simulink model "sim_v2"  (R2016b)
settings: Solver=VariableStepAuto  StartTime=0.0  StopTime=tfin  RelTol=1e-3
values from neighbouring files (symbols this model uses):
  ahat_inner_t0 = 0.5*[ahat_in1; ahat_in2]    [sim_script_circle.m]    (also in sim_script_v2.m = [ahat_in1; ahat_in2])
  ahat_outer_t0 = 0.5*[(m+m_p); c_d]    [sim_script_circle.m]    (also in sim_script_v2.m = [(m+m_p); c_d])
  c_d = 4 * 1.225 * 0.32    (= 1.568)    [sim_script_circle.m]    (also in sim_script_v2.m = 0)
  dx0 = xd(1,2)    [sim_script_circle.m]    (also in sim_script_v2.m = states(1,3))
  dz0 = zd(1,2)    [sim_script_circle.m]    (also in sim_script_v2.m = states(1,4))
  g = 9.81    [sim_script_circle.m]    (also in sim_script_v2.m)
  Gamma = 2 * diag([1, 1])    [sim_script_circle.m]    (also in sim_script_v2.m)
  Gamma_out = 0.2 * diag([1, 1])    [sim_script_circle.m]    (also in sim_script_v2.m)
  k_th = 0.2    [sim_script_circle.m]    (also in sim_script_v2.m)
  k_x = 6    [sim_script_circle.m]    (also in sim_script_v2.m)
  k_z = 6    [sim_script_circle.m]    (also in sim_script_v2.m)
  l = 0.5    [sim_script_circle.m]    (also in sim_script_v2.m)
  lambda = 3    [sim_script_circle.m]    (also in sim_script_v2.m)
  lambda_in = 6    [sim_script_circle.m]    (also in sim_script_v2.m)
  m = 3    [sim_script_circle.m]    (also in sim_script_v2.m)
  Phi_th = 0.1    [sim_script_circle.m]    (also in sim_script_v2.m)
  Phi_x = 0.4    [sim_script_circle.m]    (also in sim_script_v2.m)
  Phi_z = 0.4    [sim_script_circle.m]    (also in sim_script_v2.m)
  plan_mass = 1    [sim_script_circle.m]    (also in sim_script_v2.m = 5)
  th0 = -atan2(xd(1,3),zd(1,3)+g)    [sim_script_circle.m]    (also in sim_script_v2.m = -atan2(u(1,1)/(m+m_p),u(1,2)/(m+m_p)+g))
  Tmax = 80    [sim_script_circle.m]    (also in sim_script_v2.m)
  var_rnd = 6    [sim_script_circle.m]    (also in sim_script_v2.m)
  x0 = xd(1,1)    [sim_script_circle.m]    (also in sim_script_v2.m = states(1,1))
  z0 = zd(1,1)    [sim_script_circle.m]    (also in sim_script_v2.m = states(1,2))
libraries: cstblocks x2
settings Model: Creator=ben  LastModifiedBy=ben
settings SolverCC: ZeroCrossControl=EnableAll
settings DataIOCC: SaveOutput=off

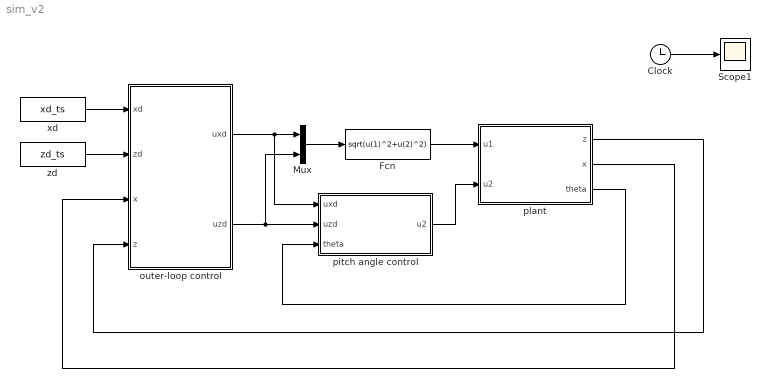
== system sim_v2 ==
  Clock : Clock
      settings: Decimation=2
  Fcn : Fcn  Expr=sqrt(u(1)^2+u(2)^2)
  Mux : Mux  Inputs=2
  Scope1 : Scope
  outer-loop control : Subsystem
  pitch angle control : Subsystem
  plant : Subsystem
  xd : FromWorkspace  VariableName=xd_ts  SampleTime=0
  zd : FromWorkspace  VariableName=zd_ts  SampleTime=0
  wires:
  xd/1 -> outer-loop control/1(xd)
  zd/1 -> outer-loop control/2(zd)
  plant/1(z) -> outer-loop control/4(z)
  plant/2(x) -> outer-loop control/3(x)
  Mux/1 -> Fcn/1
  outer-loop control/1(uxd) -> pitch angle control/1(uxd), Mux/1
  outer-loop control/2(uzd) -> pitch angle control/2(uzd), Mux/2
  Fcn/1 -> plant/1(u1)
  pitch angle control/1(u2) -> plant/2(u2)
  plant/3(theta) -> pitch angle control/3(theta)
  Clock/1 -> Scope1/1

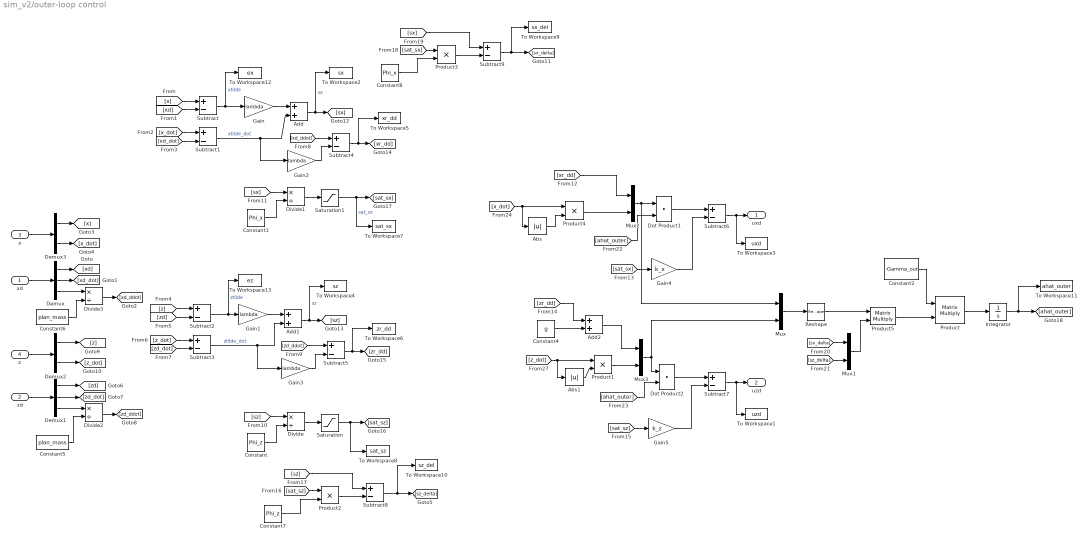
== system sim_v2/outer-loop control ==
  xd : Inport
  zd : Inport  Port=2
  x : Inport  Port=3
  z : Inport  Port=4
  Abs : Abs
  Abs1 : Abs
  Add : Sum
  Add1 : Sum
  Add2 : Sum
  Constant : Constant  Value=Phi_z
  Constant1 : Constant  Value=Phi_x
  Constant2 : Constant  Value=-Gamma_out
  Constant4 : Constant  Value=g
  Constant5 : Constant  Value=plan_mass
  Constant6 : Constant  Value=plan_mass
  Constant7 : Constant  Value=Phi_z
  Constant8 : Constant  Value=Phi_x
  Demux : Demux  Outputs=3
  Demux1 : Demux  Outputs=3
  Demux2 : Demux  Outputs=2
  Demux3 : Demux  Outputs=2
  Divide{,1..3} (4 alike) : Product  Inputs=*/
  Dot Product1 : DotProduct  InputSameDT=on  OutDataTypeStr=Inherit: Inherit via internal rule
  Dot Product2 : DotProduct  InputSameDT=on  OutDataTypeStr=Inherit: Inherit via internal rule
  Gain{,1..3} (4 alike) : Gain  Gain=lambda
  Gain4 : Gain  Gain=k_x
  Gain5 : Gain  Gain=k_z
  Integrator : Integrator  InitialCondition=ahat_outer_t0
  Mux : Mux  Inputs=[2 2]
  Mux1 : Mux  Inputs=2
  Mux2 : Mux  Inputs=2
  Mux3 : Mux  Inputs=2
  Product : Product  Multiplication=Matrix(*)
  Product{1..4} (4 alike) : Product
  Product5 : Product  Multiplication=Matrix(*)
  Reshape : Reshape  OutputDimensionality=Customize  OutputDimensions=[2,2]
  Saturation : Saturate  UpperLimit=1  LowerLimit=-1
  Saturation1 : Saturate  UpperLimit=1  LowerLimit=-1
  Subtract{,1..9} (10 alike) : Sum  Inputs=+-
  To Workspace1 : ToWorkspace  VariableName=uzd  SampleTime=-1
  To Workspace10 : ToWorkspace  VariableName=sz_del  SampleTime=-1
  To Workspace11 : ToWorkspace  VariableName=ahat_outer  SampleTime=-1
  To Workspace12 : ToWorkspace  VariableName=ex  SampleTime=-1
  To Workspace13 : ToWorkspace  VariableName=ez  SampleTime=-1
  To Workspace2 : ToWorkspace  VariableName=sx  SampleTime=-1
  To Workspace3 : ToWorkspace  VariableName=uxd  SampleTime=-1
  To Workspace4 : ToWorkspace  VariableName=sz  SampleTime=-1
  To Workspace5 : ToWorkspace  VariableName=xr_dd  SampleTime=-1
  To Workspace6 : ToWorkspace  VariableName=zr_dd  SampleTime=-1
  To Workspace7 : ToWorkspace  VariableName=sat_sx  SampleTime=-1
  To Workspace8 : ToWorkspace  VariableName=sat_sz  SampleTime=-1
  To Workspace9 : ToWorkspace  VariableName=sx_del  SampleTime=-1
  uxd : Outport
  uzd : Outport  Port=2
  wires:
  xd/1 -> Demux/1
  zd/1 -> Demux1/1
  z/1 -> Demux2/1
  x/1 -> Demux3/1
  Subtract/1 -> To Workspace12/1, Gain/1  "xtilde"
  Subtract1/1 -> Gain2/1, Add/2  "xtilde_dot"
  Gain/1 -> Add/1
  Add/1 -> To Workspace2/1, [sx]  "sx"
  Subtract2/1 -> To Workspace13/1, Gain1/1  "ztilde"
  Subtract3/1 -> Gain3/1, Add1/2  "ztilde_dot"
  Add1/1 -> To Workspace4/1, [sz]  "sz"
  Demux/1 -> [xd]
  Demux/2 -> [xd_dot]
  Demux3/1 -> [x]
  Demux3/2 -> [x_dot]
  Divide2/1 -> [zd_ddot]
  Demux1/2 -> [zd_dot]
  Demux1/1 -> [zd]
  Demux2/2 -> [z_dot]
  Demux2/1 -> [z]
  [x] -> Subtract/1
  [xd] -> Subtract/2
  [x_dot] -> Subtract1/1
  [xd_dot] -> Subtract1/2
  [z] -> Subtract2/1
  [zd] -> Subtract2/2
  [z_dot] -> Subtract3/1
  [zd_dot] -> Subtract3/2
  [xd_ddot] -> Subtract4/1
  Subtract4/1 -> To Workspace5/1, [xr_dd]
  Gain1/1 -> Add1/1
  Gain2/1 -> Subtract4/2
  Gain3/1 -> Subtract5/2
  [zd_ddot] -> Subtract5/1
  Subtract5/1 -> To Workspace6/1, [zr_dd]
  Divide/1 -> Saturation/1
  [sz] -> Divide/1
  Constant/1 -> Divide/2
  Saturation/1 -> [sat_sz], To Workspace8/1
  Divide1/1 -> Saturation1/1
  [sx] -> Divide1/1
  Constant1/1 -> Divide1/2
  Saturation1/1 -> To Workspace7/1, [sat_sx]  "sat_sx"
  [xr_dd] -> Mux2/1
  [ahat_outer] -> Dot Product1/2
  Dot Product1/1 -> Subtract6/1
  Gain4/1 -> Subtract6/2
  Subtract6/1 -> To Workspace3/1, uxd/1
  [sat_sx] -> Gain4/1
  [zr_dd] -> Add2/1
  [ahat_outer] -> Dot Product2/2
  Dot Product2/1 -> Subtract7/1
  Gain5/1 -> Subtract7/2
  [sat_sz] -> Gain5/1
  Subtract7/1 -> To Workspace1/1, uzd/1
  Add2/1 -> Mux3/1
  Constant4/1 -> Add2/2
  Constant5/1 -> Divide2/2
  Demux1/3 -> Divide2/1
  Divide3/1 -> [xd_ddot]
  Constant6/1 -> Divide3/2
  Demux/3 -> Divide3/1
  Product2/1 -> Subtract8/2
  Constant7/1 -> Product2/2
  [sat_sz] -> Product2/1
  [sz] -> Subtract8/1
  Subtract8/1 -> To Workspace10/1, [sz_delta]
  Product3/1 -> Subtract9/2
  Constant8/1 -> Product3/2
  [sat_sx] -> Product3/1
  [sx] -> Subtract9/1
  Subtract9/1 -> To Workspace9/1, [sx_delta]
  [sx_delta] -> Mux1/1
  [sz_delta] -> Mux1/2
  Mux/1 -> Reshape/1
  Mux1/1 -> Product5/2
  Product/1 -> Integrator/1
  Integrator/1 -> To Workspace11/1, [ahat_outer]
  Mux2/1 -> Mux/1, Dot Product1/1
  [x_dot] -> Product4/1, Abs/1
  Abs/1 -> Product4/2
  Mux3/1 -> Dot Product2/1, Mux/2
  Product1/1 -> Mux3/2
  Abs1/1 -> Product1/2
  [z_dot] -> Product1/1, Abs1/1
  Reshape/1 -> Product5/1
  Constant2/1 -> Product/1
  Product5/1 -> Product/2
  Product4/1 -> Mux2/2

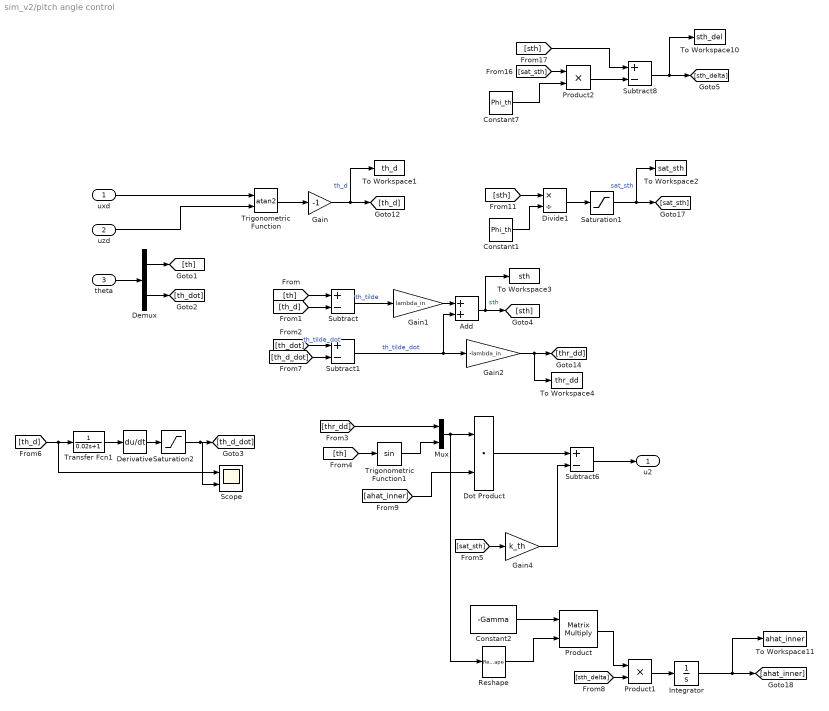
== system sim_v2/pitch angle control ==
  uxd : Inport
  uzd : Inport  Port=2
  theta : Inport  Port=3
  Add : Sum
  Constant1 : Constant  Value=Phi_th
  Constant2 : Constant  Value=-Gamma
  Constant7 : Constant  Value=Phi_th
  Demux : Demux  Outputs=2
  Derivative : Derivative
  Divide1 : Product  Inputs=*/
  Dot Product : DotProduct  InputSameDT=on  OutDataTypeStr=Inherit: Inherit via internal rule
  Gain : Gain  Gain=-1
  Gain1 : Gain  Gain=lambda_in
  Gain2 : Gain  Gain=-lambda_in
  Gain4 : Gain  Gain=k_th
  Integrator : Integrator  InitialCondition=ahat_inner_t0
  Mux : Mux  Inputs=2
  Product : Product  Multiplication=Matrix(*)
  Product1 : Product
  Product2 : Product
  Reshape : Reshape  OutputDimensionality=Column vector (2-D)
  Saturation1 : Saturate  UpperLimit=1  LowerLimit=-1
  Saturation2 : Saturate  UpperLimit=1  LowerLimit=-1
  Scope : Scope  NumInputPorts=2
  Subtract{,1,6,8} (4 alike) : Sum  Inputs=+-
  To Workspace1 : ToWorkspace  VariableName=th_d  SampleTime=-1
  To Workspace10 : ToWorkspace  VariableName=sth_del  SampleTime=-1
  To Workspace11 : ToWorkspace  VariableName=ahat_inner  SampleTime=-1
  To Workspace2 : ToWorkspace  VariableName=sat_sth  SampleTime=-1
  To Workspace3 : ToWorkspace  VariableName=sth  SampleTime=-1
  To Workspace4 : ToWorkspace  VariableName=thr_dd  SampleTime=-1
  Transfer Fcn1 : TransferFcn  Denominator=[0.02 1]
  Trigonometric Function : Trigonometry  Operator=atan2
  Trigonometric Function1 : Trigonometry
  u2 : Outport
  wires:
  uxd/1 -> Trigonometric Function/1
  uzd/1 -> Trigonometric Function/2
  Trigonometric Function/1 -> Gain/1
  Gain/1 -> To Workspace1/1, [th_d]  "th_d"
  Demux/1 -> [th]
  theta/1 -> Demux/1
  Demux/2 -> [th_dot]
  Subtract/1 -> Gain1/1  "th_tilde"
  Subtract1/1 -> Add/2, Gain2/1  "th_tilde_dot"
  Gain1/1 -> Add/1
  Add/1 -> To Workspace3/1, [sth]  "sth"
  [th] -> Subtract/1
  [th_d] -> Subtract/2
  Gain2/1 -> To Workspace4/1, [thr_dd]
  [thr_dd] -> Mux/1
  Trigonometric Function1/1 -> Mux/2
  [th] -> Trigonometric Function1/1
  Mux/1 -> Dot Product/1, Reshape/1
  [ahat_inner] -> Dot Product/2
  Divide1/1 -> Saturation1/1
  [sth] -> Divide1/1
  Constant1/1 -> Divide1/2
  Saturation1/1 -> To Workspace2/1, [sat_sth]  "sat_sth"
  Gain4/1 -> Subtract6/2
  Subtract6/1 -> u2/1
  [sat_sth] -> Gain4/1
  Dot Product/1 -> Subtract6/1
  Derivative/1 -> Saturation2/1
  [th_d_dot] -> Subtract1/2
  [th_dot] -> Subtract1/1  "th_tilde_dot"
  Saturation2/1 -> Scope/2, [th_d_dot]
  [th_d] -> Transfer Fcn1/1, Scope/1
  Product1/1 -> Integrator/1
  Integrator/1 -> To Workspace11/1, [ahat_inner]
  Product2/1 -> Subtract8/2
  Constant7/1 -> Product2/2
  [sat_sth] -> Product2/1
  [sth] -> Subtract8/1
  Subtract8/1 -> To Workspace10/1, [sth_delta]
  Constant2/1 -> Product/1
  [sth_delta] -> Product1/2
  Product/1 -> Product1/1
  Reshape/1 -> Product/2
  Transfer Fcn1/1 -> Derivative/1

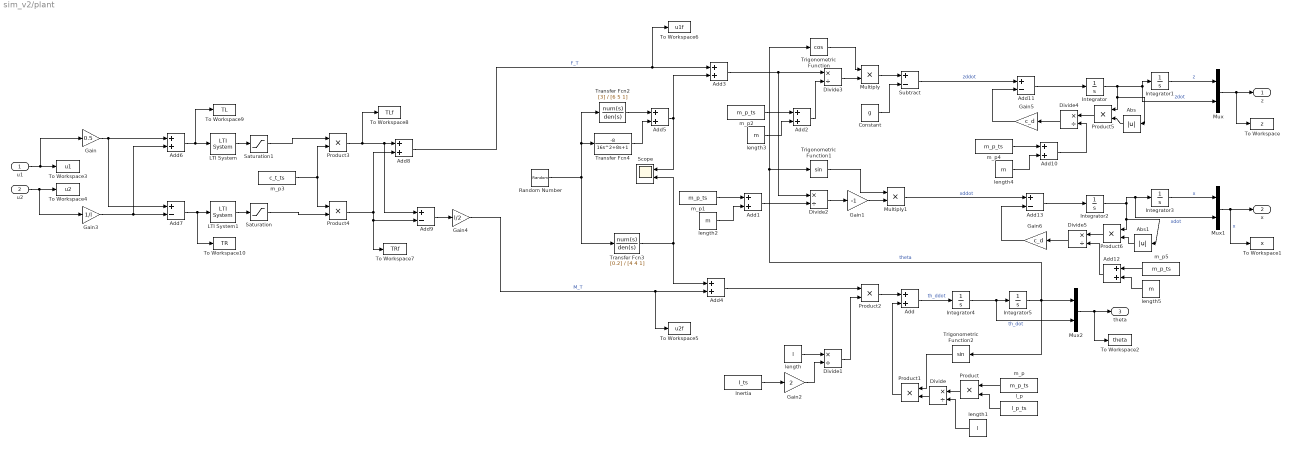
== system sim_v2/plant ==
  u1 : Inport
  u2 : Inport  Port=2
  Abs : Abs
  Abs1 : Abs
  Add{,1..6,8,10,12} (10 alike) : Sum
  Add{7,9,11,13} (4 alike) : Sum  Inputs=+-
  Constant : Constant  Value=g
  Divide{,1..5} (6 alike) : Product  Inputs=*/
  Gain : Gain  Gain=0.5
  Gain1 : Gain  Gain=-1
  Gain2 : Gain  Gain=2
  Gain3 : Gain  Gain=1/l
  Gain4 : Gain  Gain=l/2
  Gain5 : Gain  Gain=c_d
  Gain6 : Gain  Gain=c_d
  Inertia : FromWorkspace  VariableName=I_ts  SampleTime=0
  Integrator : Integrator  InitialCondition=dz0
  Integrator1 : Integrator  InitialCondition=z0
  Integrator2 : Integrator  InitialCondition=dx0
  Integrator3 : Integrator  InitialCondition=x0
  Integrator4 : Integrator
  Integrator5 : Integrator  InitialCondition=th0
  LTI System : cstblocks/LTI System  sys=tf_act  IC=[]
  LTI System1 : cstblocks/LTI System  sys=tf_act  IC=[]
  Multiply : Product  Inputs=**
  Multiply1 : Product  Inputs=**
  Mux : Mux  Inputs=2
  Mux1 : Mux  Inputs=2
  Mux2 : Mux  Inputs=2
  Product{,1..6} (7 alike) : Product
  Random Number : RandomNumber  Variance=var_rnd  SampleTime=0.1
  Saturation : Saturate  UpperLimit=Tmax  LowerLimit=0
  Saturation1 : Saturate  UpperLimit=Tmax  LowerLimit=0
  Scope : Scope  NumInputPorts=2
  Subtract : Sum  Inputs=+-
  To Workspace : ToWorkspace  VariableName=z  SampleTime=-1
  To Workspace1 : ToWorkspace  VariableName=x  SampleTime=-1
  To Workspace10 : ToWorkspace  VariableName=TR  SampleTime=-1
  To Workspace2 : ToWorkspace  VariableName=theta  SampleTime=-1
  To Workspace3 : ToWorkspace  VariableName=u1  SampleTime=-1
  To Workspace4 : ToWorkspace  VariableName=u2  SampleTime=-1
  To Workspace5 : ToWorkspace  VariableName=u2f  SampleTime=-1
  To Workspace6 : ToWorkspace  VariableName=u1f  SampleTime=-1
  To Workspace7 : ToWorkspace  VariableName=TRf  SampleTime=-1
  To Workspace8 : ToWorkspace  VariableName=TLf  SampleTime=-1
  To Workspace9 : ToWorkspace  VariableName=TL  SampleTime=-1
  Transfer Fcn2 : TransferFcn  Numerator=[3]  Denominator=[6 5 1]
  Transfer Fcn3 : TransferFcn  Numerator=[0.2]  Denominator=[4 4 1]
  Transfer Fcn4 : TransferFcn  Numerator=[-8]  Denominator="[16 8  1]"
  Trigonometric Function : Trigonometry  Operator=cos
  Trigonometric Function1 : Trigonometry
  Trigonometric Function2 : Trigonometry
  l_p : FromWorkspace  VariableName=l_p_ts  SampleTime=0
  length : Constant  Value=l
  length1 : Constant  Value=l
  length{2..5} (4 alike) : Constant  Value=m
  m_p{,1..2,4..5} (5 alike) : FromWorkspace  VariableName=m_p_ts  SampleTime=0
  m_p3 : FromWorkspace  VariableName=c_t_ts  SampleTime=0
  z : Outport
  x : Outport  Port=2
  theta : Outport  Port=3
  wires:
  Constant/1 -> Subtract/2
  Subtract/1 -> Add11/1  "zddot"
  Integrator5/1 -> Mux2/1, Trigonometric Function2/1, Trigonometric Function1/1, Trigonometric Function/1  "theta"
  Multiply/1 -> Subtract/1
  Add/1 -> Integrator4/1  "th_ddot"
  Divide3/1 -> Multiply/2
  Trigonometric Function/1 -> Multiply/1
  Integrator4/1 -> Mux2/2, Integrator5/1  "th_dot"
  u2/1 -> Gain3/1, To Workspace4/1
  Gain1/1 -> Multiply1/2
  Trigonometric Function1/1 -> Multiply1/1
  Multiply1/1 -> Add13/1  "xddot"
  Mux1/1 -> To Workspace1/1, x/1  "x"
  Product1/1 -> Add/2
  Trigonometric Function2/1 -> Product1/1
  Integrator/1 -> Abs/1, Product5/1, Integrator1/1, Mux/2  "zdot"
  Integrator1/1 -> Mux/1  "z"
  Mux/1 -> To Workspace/1, z/1
  Integrator3/1 -> Mux1/1  "x"
  Mux2/1 -> To Workspace2/1, theta/1
  m_p/1 -> Product/1
  l_p/1 -> Product/2
  Product/1 -> Divide/1
  length1/1 -> Divide/2
  Divide/1 -> Product1/2
  Product2/1 -> Add/1
  length/1 -> Divide1/1
  Gain2/1 -> Divide1/2
  Inertia/1 -> Gain2/1
  Divide1/1 -> Product2/2
  Divide2/1 -> Gain1/1
  Add1/1 -> Divide2/2
  m_p1/1 -> Add1/1
  length2/1 -> Add1/2
  m_p2/1 -> Add2/1
  length3/1 -> Add2/2
  Add2/1 -> Divide3/2
  u1/1 -> Gain/1, To Workspace3/1
  Add3/1 -> Divide2/1, Divide3/1
  Add5/1 -> Add3/2, Scope/1
  Add4/1 -> Product2/1
  Transfer Fcn3/1 -> Scope/2, Add4/1
  Random Number/1 -> Transfer Fcn4/1, Transfer Fcn2/1, Transfer Fcn3/1
  Transfer Fcn2/1 -> Add5/1
  Transfer Fcn4/1 -> Add5/2
  Gain/1 -> Add7/1, Add6/1
  Gain3/1 -> Add7/2, Add6/2
  Add7/1 -> LTI System1/1, To Workspace10/1
  Add6/1 -> LTI System/1, To Workspace9/1
  LTI System/1 -> Saturation1/1
  LTI System1/1 -> Saturation/1
  Add9/1 -> Gain4/1
  Product4/1 -> Add8/2, To Workspace7/1, Add9/2
  Product3/1 -> To Workspace8/1, Add9/1, Add8/1
  Add8/1 -> Add3/1, To Workspace6/1  "F_T"
  Gain4/1 -> Add4/2, To Workspace5/1  "M_T"
  m_p3/1 -> Product4/1, Product3/2
  Saturation1/1 -> Product3/1
  Saturation/1 -> Product4/2
  m_p4/1 -> Add10/1
  length4/1 -> Add10/2
  Add10/1 -> Divide4/2
  Divide4/1 -> Gain5/1
  Gain5/1 -> Add11/2
  Add11/1 -> Integrator/1
  Product5/1 -> Divide4/1
  Abs/1 -> Product5/2
  Integrator2/1 -> Mux1/2, Integrator3/1, Abs1/1, Product6/1  "xdot"
  m_p5/1 -> Add12/1
  length5/1 -> Add12/2
  Add12/1 -> Divide5/2
  Divide5/1 -> Gain6/1
  Gain6/1 -> Add13/2
  Product6/1 -> Divide5/1
  Abs1/1 -> Product6/2
  Add13/1 -> Integrator2/1
